simulink model "phase4_attitude_control"  (R2017b)
settings: Solver=VariableStepAuto  StartTime=0.0  StopTime=0.4  RelTol=1e-3
values from neighbouring files (symbols this model uses):
  c = 1.140*10^-7    (= 1.14e-07)    [run_this_and_plot.m]
  Ix = 4.856*10^(-3)    (= 0.004856)    [run_this_and_plot.m]
  Iy = 4.856*10^(-3)    (= 0.004856)    [run_this_and_plot.m]
  Iz = 8.801*10^(-3)    (= 0.008801)    [run_this_and_plot.m]
  k = 2.980*10^-6    (= 2.98e-06)    [run_this_and_plot.m]
  l = 0.225    [run_this_and_plot.m]
settings Model: Creator=Administrator  LastModifiedBy=chenjiasheng
settings CodeAppCC: StateflowObjectComments=on

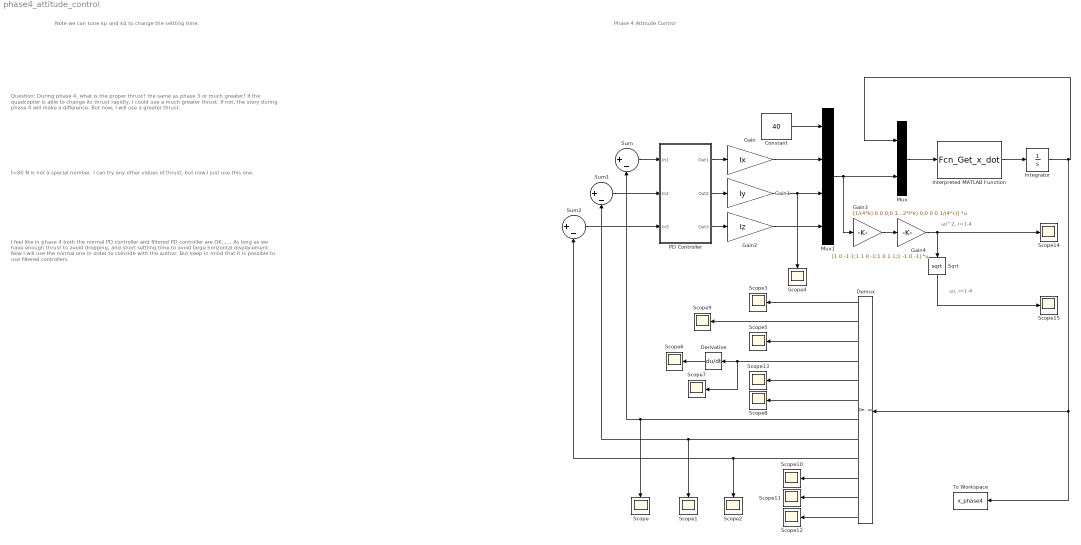
== system phase4_attitude_control ==
  note: f=80 N is not a special number. I can try any other values of thrust, but now I just use this one.
  note: Note we can tune kp and kd to change the settling time.
  note: I feel like in phase 4 both the normal PD controller and filtered PD controller are OK......
      | As long as we have enough thrust to avoid dropping, and short settling time to avoid large horizontal displacement.
      | Now I will use the normal one in order to coincide with the author. But keep in mind that it is possible to use filtered controllers.
  note: Question: During phase 4, what is the proper thrust? the same as phase 3 or much greater?
      | If the quadcopter is able to change its thrust rapidly, I could use a much greater thrust. If not, the story during phase 4 will make a difference. But now, I will use a greater thrust.
  note: Phase 4 Attitude Control
  note: ωi^2, i=1-4
  note: ωi, i=1-4
  Constant : Constant  Value=40
  Demux : Demux  Outputs=12
  Derivative : Derivative
  Gain : Gain  Gain=Ix
  Gain1 : Gain  Gain=Iy
  Gain2 : Gain  Gain=Iz
  Gain3 : Gain  Gain=[1/(4*k) 0 0 0;0 1/(2*l*k) 0 0;0 0 1/(2*l*k) 0;0 0 0 1/(4*c)]  Multiplication=Matrix(K*u) (u vector)
  Gain4 : Gain  Gain=[1 0 -1 1;1 1 0 -1;1 0 1 1;1 -1 0 -1]  Multiplication=Matrix(K*u) (u vector)
  Integrator : Integrator  InitialCondition=x_phase3(end,:)
  Interpreted MATLAB Function : MATLABFcn  MATLABFcn=Fcn_Get_x_dot
  Mux : Mux  Inputs=2
  Mux1 : Mux
  PD Controller : Subsystem
  Scope{,1..15} (16 alike) : Scope
  Sqrt : Sqrt  SaturateOnIntegerOverflow=on
  Sum : Sum  Inputs=|+-
  Sum1 : Sum  Inputs=|+-
  Sum2 : Sum  Inputs=|+-
  To Workspace : ToWorkspace  VariableName=x_phase4  SampleTime=0.01
  wires:
  Mux/1 -> Interpreted MATLAB Function/1
  Interpreted MATLAB Function/1 -> Integrator/1
  Integrator/1 -> To Workspace/1, Demux/1, Mux/1
  Mux1/1 -> Mux/2, Gain3/1
  Gain/1 -> Mux1/2
  Gain1/1 -> Scope4/1, Mux1/3
  Gain2/1 -> Mux1/4
  Demux/7 -> Scope/1, Sum/2
  Demux/8 -> Sum1/2, Scope1/1
  Demux/9 -> Scope2/1, Sum2/2
  Demux/3 -> Scope5/1
  Demux/4 -> Scope7/1, Derivative/1
  Demux/6 -> Scope8/1
  Derivative/1 -> Scope6/1
  Demux/1 -> Scope3/1
  Constant/1 -> Mux1/1
  Demux/2 -> Scope9/1
  Demux/10 -> Scope10/1
  Demux/11 -> Scope11/1
  Demux/12 -> Scope12/1
  Demux/5 -> Scope13/1
  Gain4/1 -> Scope14/1, Sqrt/1
  Gain3/1 -> Gain4/1
  Sqrt/1 -> Scope15/1
  PD Controller/1(Out1) -> Gain/1
  PD Controller/2(Out2) -> Gain1/1
  Sum/1 -> PD Controller/1(In1)
  PD Controller/3(Out3) -> Gain2/1
  Sum1/1 -> PD Controller/2(In2)
  Sum2/1 -> PD Controller/3(In3)

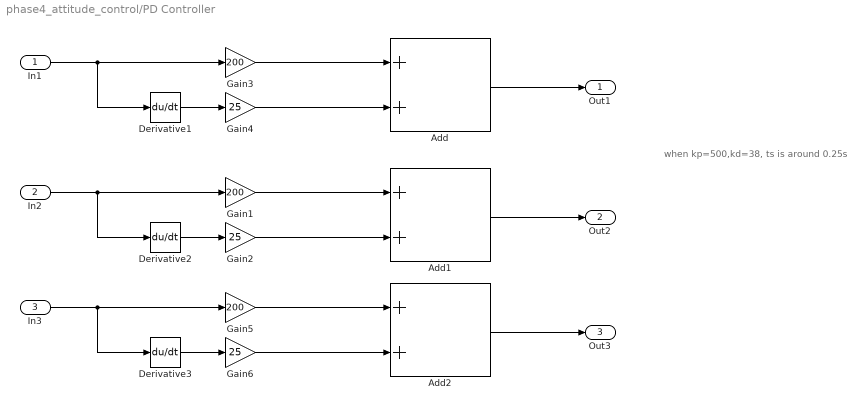
== system phase4_attitude_control/PD Controller ==
  note: when kp=500,kd=38, ts is around 0.25s
  In1 : Inport
  In2 : Inport  Port=2
  In3 : Inport  Port=3
  Add : Sum
  Add1 : Sum
  Add2 : Sum
  Derivative1 : Derivative
  Derivative2 : Derivative
  Derivative3 : Derivative
  Gain1 : Gain  Gain=200
  Gain2 : Gain  Gain=25
  Gain3 : Gain  Gain=200
  Gain4 : Gain  Gain=25
  Gain5 : Gain  Gain=200
  Gain6 : Gain  Gain=25
  Out1 : Outport
  Out2 : Outport  Port=2
  Out3 : Outport  Port=3
  wires:
  Gain3/1 -> Add/1
  In1/1 -> Derivative1/1, Gain3/1
  Gain4/1 -> Add/2
  Derivative1/1 -> Gain4/1
  Add/1 -> Out1/1
  Add1/1 -> Out2/1
  Derivative2/1 -> Gain2/1
  Gain2/1 -> Add1/2
  In2/1 -> Gain1/1, Derivative2/1
  Gain1/1 -> Add1/1
  Gain5/1 -> Add2/1
  In3/1 -> Derivative3/1, Gain5/1
  Gain6/1 -> Add2/2
  Derivative3/1 -> Gain6/1
  Add2/1 -> Out3/1
